simulink library "Inverter_CONF"  (R2016b)
settings: Solver=ode45  StartTime=0.0  StopTime=10.0  RelTol=1e-3  EnableMultiTasking=on
undefined symbols (not defined in the file): path_carnot
libraries: carnot x1
settings Model: Creator=srrt  LastModifiedBy=drhf
settings DataIOCC: LimitDataPoints=on  SaveFormat=Array
settings OptimizationCC: LifeSpan=inf
settings DebuggingCC: UnderspecifiedInitializationDetection=Classic  MergeDetectMultiDrivingBlocksExec=none  SolverPrmCheckMsg=warning  SFUnexpectedBacktrackingDiag=warning  SFNoUnconditionalDefaultTransitionDiag=warning  SFExecutionAtInitializationDiag=none
settings HardwareCC: ProdBitPerPointer=32  ProdBitPerSizeT=32  ProdBitPerPtrDiffT=32  ProdLargestAtomicFloat=None  ProdIntDivRoundTo=Undefined  ProdEndianess=Unspecified  ProdWordSize=32  ProdHWDeviceType=32-bit Generic
settings ModelReferenceCC: PropagateSignalLabelsOutOfModel=off
settings GRTTargetCC: TargetLangStandard=C89/C90 (ANSI)  GeneratePreprocessorConditionals=Disable all
settings ConfigComp: CovMetricSettings=dw  CovHtmlReporting=on  CovSaveCumulativeToWorkspaceVar=on  CovSaveSingleToWorkspaceVar=on  CovExternalEMLEnable=off  CovSFcnEnable=off

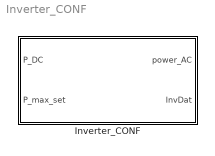
== system Inverter_CONF ==
  Inverter_CONF : Subsystem  mask(Configurated Inverter){PathName=fullfile(path_carnot('libsl'), 'Source','Electric_Generator','Inverter_CONF','parameter_set'), FileName='SMA_SB2_5_VL40.mat', userPath=off, userParam=off, Pacnom=2500, overload=1, PstepsEta=[0 0.1 0.2 0.25 0.3 0.5 0.75 1], Eta=[0 0.948 0.966 0.969 0.97 0.972 0.97 0.967], P_standby=2}
      mask prompts: PathName "Path"; FileName "Parameter set"; userPath "Edit path and name of parameter set"; userParam "User defined parameters"; Pacnom "nominal power in W"; overload "overload (0.5 ...1.5)"; PstepsEta "steps for efficiency (0..1..overload)"; Eta "efficiency (0..1)"; P_standby "Standby power consumption in W"
      mask help:
      | This block considers the eficiency of the inverter based on
      | - eta euro [1]
      | In the simple model the efficieny of the inverter is assumed to be constant.
      | This block uses predefined parameter sets.
      mask init:
      | % callback to set parameters of model
      | [ok, param] = CarnotCallbacks_InverterConf('SetParameters',gcbh,PathName,FileName);
      mask Help: web(fullfile(path_carnot('help'),'Inverter_CONF.html'),'-helpbrowser')
      mask Callback userPath: [ok, param] = CarnotCallbacks_InverterConf('UserEdit',gcbh);
      mask Callback userParam: [ok, param] = CarnotCallbacks_InverterConf('UserEdit',gcbh);
      mask TypeOptions Pacnom: Inverter/P0
      mask TypeOptions overload: Inverter/ol
      mask TypeOptions PstepsEta: Inverter/power_steps
      mask TypeOptions Eta: Inverter/eta_steps
      mask TypeOptions P_standby: Inverter/standby
      mask DialogControl Control2 Prompt: Carnot public data
      mask DialogControl Control2 Callback: [ok, file] = CarnotCallbacks_InverterConf('GetFilename',gcbh,'public');
      mask DialogControl Control3 Prompt: Carnot internal data
      mask DialogControl Control3 Callback: [ok, file] = CarnotCallbacks_InverterConf('GetFilename',gcbh,'internal');
      mask DialogControl Control4 Prompt: Selected path
      mask DialogControl Control4 Callback: [ok, file] = CarnotCallbacks_InverterConf('GetFilename',gcbh,'selected');
      mask DialogControl Control5 Prompt: Save in Carnot internal data
      mask DialogControl Control5 Callback: [ok, param] = CarnotCallbacks_InverterConf('SaveFilename',gcbh,'internal','IVRT');
      mask DialogControl Control6 Prompt: Save in selected path
      mask DialogControl Control6 Callback: [ok, param] = CarnotCallbacks_InverterConf('SaveFilename',gcbh,'selected','IVRT');
      mask Display:
      | %plot([0,0],[0,1],[-0.5,1.5],[0,0],power_steps, eta_steps)
      | plot(-40,0,140,100,[90,10,90,90,10,10],[10,90,90,10,10,90],[40,20],[40,40],[40,20],[30,30],[88,84,75,64,55,50],[70,60,60,80,80,70])

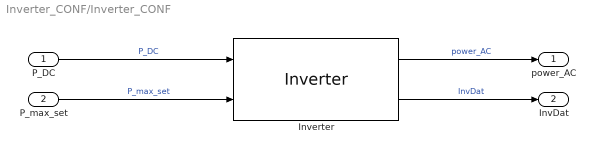
== system Inverter_CONF/Inverter_CONF ==
  P_DC : Inport
  P_max_set : Inport  Port=2
  Inverter : carnot/Source/Electric_Generator/Inverter  P0=Pacnom  ol=overload  power_steps=PstepsEta  eta_steps=Eta  standby=P_standby
  power_AC : Outport
  InvDat : Outport  Port=2
  wires:
  Inverter/2 -> InvDat/1  "InvDat"
  Inverter/1 -> power_AC/1  "power_AC"
  P_max_set/1 -> Inverter/2  "P_max_set"
  P_DC/1 -> Inverter/1  "P_DC"
